simulink model "PlanerizerTest03"  (R2023a)
settings: Solver=FixedStepAuto  StartTime=0.0  StopTime=inf  FixedStep=0.005  RelTol=1e-3
libraries: speedgoatlib_IO691 x6, canmsglib x6, slrealtimeutilitieslib x2
settings Model: SimulationMode=external  NumberOfSteps=2  ExtModeEnableFloating=off  Creator=celwe  LastModifiedBy=johna
settings SolverCC: ConcurrentTasks=on  PositivePriorityOrder=on
settings OptimizationCC: BlockReduction=off  OptimizeBlockIOStorage=off
settings DebuggingCC: TasksWithSamePriorityMsg=none  UnconnectedInputMsg=warning  UnconnectedOutputMsg=warning  UnconnectedLineMsg=warning
settings HardwareCC: ProdBitPerLong=64  ProdLongLongMode=on  ProdHWDeviceType=Intel->x86-64 (Linux 64)
settings ModelReferenceCC: EnableRefExpFcnMdlSchedulingChecks=on
settings RTWCC: Description=Simulink Real-Time  SystemTargetFile=slrealtime.tlc  TemplateMakefile=slrealtime_default_tmf  Toolchain=Simulink Real-Time Toolchain  BuildConfiguration=Faster Runs  CodeExecutionProfiling=on  TargetLang=C++  DLArmComputeVersion=19.05

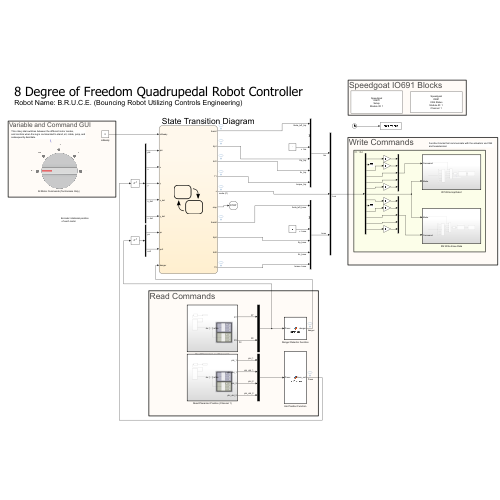
[thumbnail: Simulink's stored preview of the top-level diagram]
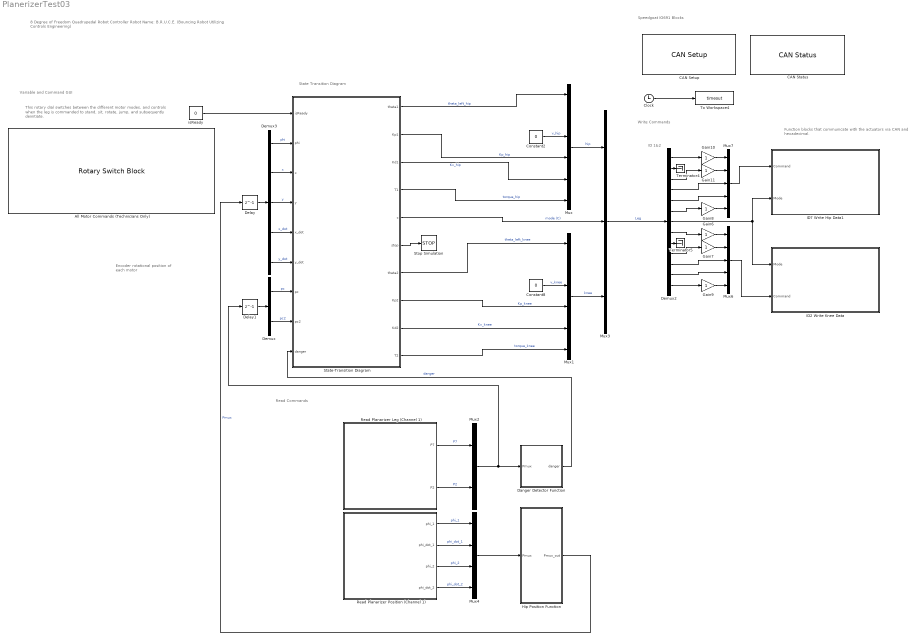
== system PlanerizerTest03 ==
  note: Variable and Command GUI
  note: 8 Degree of Freedom Quadrupedal Robot Controller
      | Robot Name: B.R.U.C.E. (Bouncing Robot Utilizing Controls Engineering)
  note: Encoder rotational position
      |  of each motor
  note: This rotary dial switches between the different motor modes,
      | and controls when the leg is commanded to stand, sit, rotate, jump, and
      | subsequently deinitiate.
  note: ID 1&2
  note: Function blocks that communicate with the actuators via CAN
      | and hexadecimal.
  note: Speedgoat IO691 Blocks
  note: Read Commands
  note: Write Commands
  note: State Transition Diagram
  "All Motor Commands (Technicians Only) " : RotarySwitchBlock
      settings: Values={{'Zeroing', 'Initiated', 'Stand', 'Sit', 'deinit'}, [0 1 2 3 4]}
  "CAN Setup " : speedgoatlib_IO691/Legacy/CAN Setup   moduletype=IO691  id=1  pciSlot=-1  chn1=CAN (HS)  chn2=CAN (HS)  chn3=Disabled  chn4=Disabled  initStruct=[]  termStruct=[]  ArbitrationbdrChn1=1.0 MBaud  ArbitrationManbdrChn1=[2,8,31,8]  FdbdrChn1=5.0 MBaud  FdManbdrChn1=[2,2,5,2]  ArbitrationbdrChn2=1.0 MBaud  ArbitrationManbdrChn2=[2,8,31,8]  FdbdrChn2=5.0 MBaud  FdManbdrChn2=[2,2,5,2]  ArbitrationbdrChn3=1.0 MBaud  ArbitrationManbdrChn3=[2,8,31,8]  FdbdrChn3=5.0 MBaud  FdManbdrChn3=[2,2,5,2]  ArbitrationbdrChn4=1.0 MBaud  ArbitrationManbdrChn4=[2,8,31,8]  FdbdrChn4=5.0 MBaud  FdManbdrChn4=[2,2,5,2]  moduleInitValues=[691 1 -1 -1]
      settings: SourceProductName=Simulink Real-Time: Speedgoat I/O Blockset
  CAN Status : speedgoatlib_IO691/Legacy/CAN Status  moduleId=1  sampleTime=-1  channel=1  busRecovery=Off  arrayOutput=off  controllerCpuLoad=off  controllerLiveCount=off  initModeAct=off  avgBusLoad=off  receiving=off  RxQueueEmpty=off  dataOverrunRcv=off  rxBufferLevel=off  txPending=off  dataOverrunTx=off  txBufferLevel=off  errWarnLimit=off  errPassLimit=off  errBusOff=off  busRecoveryCounter=off  busCouplingErr=off  transceiverErr=off  opMode=off  brp=off  timeSegment1=off  timeSegment2=off  synchronisationJumpWidth=off  dataTSEG1=off  dataTSEG2=off  dataSJW=off  moduleType=691  qtyStatBlk=1  ptIdx=0  isFDMod=0
      settings: SourceProductName=Simulink Real-Time: Speedgoat I/O Blockset
  Clock : Clock
  Constant2 : Constant  Value=0
  Constant8 : Constant  Value=0
  Danger Detector Function : MATLAB Function  TreatAsAtomicUnit=on
  Delay : Delay  DelayLength=1
  Delay1 : Delay  DelayLength=1
  Demux : Demux  Outputs=2
  Demux2 : Demux  Outputs=13
  Demux3 : Demux  Outputs=5
  Gain{6..11} (6 alike) : Gain
  Hip Position Function : MATLAB Function  TreatAsAtomicUnit=on
  ID2 Write Knee Data : Subsystem  TreatAsAtomicUnit=on
  ID7 Write Hip Data1 : Subsystem  TreatAsAtomicUnit=on
  Mux : Mux  Inputs=6
  Mux1 : Mux  Inputs=6
  Mux2 : Mux  Inputs=2
  Mux3 : Mux  Inputs=3
  Mux4 : Mux
  Mux6 : Mux  Inputs=5
  Mux7 : Mux  Inputs=5
  Read Planarizer Leg (Channel 1) : Subsystem  TreatAsAtomicUnit=on
  Read Planarizer Position (Channel 1) : Subsystem  TreatAsAtomicUnit=on
  State-Transition Diagram : Stateflow chart  TreatAsAtomicUnit=on
      settings: PortSchema="{\"entries\":[{\"content\":{\"sides\":[{\"content\":{\"connectorIds\":[\"In9\",\"In2\",\"In3\",\"In4\",\"In5\",\"In6\",\"In1\",\"In7\",\"In8\"]},\"type\":\"ConnectorPlacement.EquallySpacedRectSide\",\"uuid\":\"09499f21-f50c-4ce4-914e-8b9942bcc246\"},{\"content\":{\"connectorIds\":[\"Out2\",\"Out7\",\"Out9\",\"Out5\",\"Out4\",\"Out1\",\"Out3\",\"Out8\",\"Out10\",\"Out6\"],\"side\":\"RIGHT\"},\"type\":\"ConnectorPlacement.EquallySpacedRectSide\",\"uuid\":\"b935e908-ace3-4dfb-ad6d-08dfed6ffdb3\"},{\"content\":{\"side\":\"TOP\"},\"type\":\"ConnectorPlacement.EquallySpacedRectSide\",\"uuid\":\"4cd7c5d6-1f1f-4a1f-84b4-9b198395645e\"}]},\"type\":\"ConnectorPlacement.EquallySpacedConnector\",\"uuid\":\"2dc6a8af-05a8-4f21-87ab-6863f156f450\"}],\"packageUris\":[\"http://schema.mathworks.com/mf0/Connector/R2020b\"],\"version\":\"1.0\"}"
  Stop Simulation : Stop
  Terminator4 : Terminator
  Terminator5 : Terminator
  To Workspace4 : ToWorkspace  VariableName=timeout  SampleTime=-1
  isReady : Constant  Value=0
  wires:
  Mux/1 -> Mux3/1  "hip"
  State-Transition Diagram/7(Kp1) -> Mux/4  "Kp_hip"
  State-Transition Diagram/5(T1) -> Mux/6  "torque_hip"
  Constant8/1 -> Mux1/3  "v_knee"
  Mux1/1 -> Mux3/3  "knee"
  State-Transition Diagram/4(c) -> Mux3/2  "mode (C)"
  Mux2/1 -> Delay1/1, Danger Detector Function/1(Pmux)
  State-Transition Diagram/1(stop) -> Stop Simulation/1
  isReady/1 -> State-Transition Diagram/9(isReady)
  Clock/1 -> To Workspace4/1
  State-Transition Diagram/9(Kd1) -> Mux/5  "Kv_hip"
  Constant2/1 -> Mux/3  "v_hip"
  State-Transition Diagram/2(theta1) -> Mux/1  "theta_left_hip"
  Mux3/1 -> Demux2/1  "Leg"
  Mux7/1 -> ID7 Write Hip Data1/1(Command)
  Mux6/1 -> ID2 Write Knee Data/2(Command)
  Read Planarizer Leg (Channel 1)/2(P2) -> Mux2/2  "P2"
  Demux/2 -> State-Transition Diagram/7(pc2)  "pc2"
  Demux/1 -> State-Transition Diagram/1(pc)  "pc"
  Demux2/7 -> ID7 Write Hip Data1/2(Mode), ID2 Write Knee Data/1(Mode)
  Demux2/4 -> Mux7/3
  Demux2/10 -> Gain7/1
  Demux2/6 -> Gain8/1
  Demux2/5 -> Mux7/4
  Demux2/11 -> Mux6/3
  Demux2/3 -> Gain11/1
  Demux2/12 -> Mux6/4
  Gain11/1 -> Mux7/2
  Gain10/1 -> Mux7/1
  Gain7/1 -> Mux6/2
  Demux2/13 -> Gain9/1
  Gain9/1 -> Mux6/5
  Gain8/1 -> Mux7/5
  Gain6/1 -> Mux6/1
  State-Transition Diagram/3(theta2) -> Mux1/1  "theta_left_knee"
  State-Transition Diagram/10(Kd2) -> Mux1/5  "Kv_knee"
  State-Transition Diagram/6(T2) -> Mux1/6  "torque_knee"
  State-Transition Diagram/8(Kp2) -> Mux1/4  "Kp_knee"
  Read Planarizer Leg (Channel 1)/1(P7) -> Mux2/1  "P7"
  Danger Detector Function/1(danger) -> State-Transition Diagram/8(danger)  "danger"
  Demux2/2 -> Terminator4/1
  Demux2/1 -> Gain10/1
  Demux2/9 -> Terminator5/1
  Demux2/8 -> Gain6/1
  Read Planarizer Position (Channel 1)/1(phi_1) -> Mux4/1  "phi_1"
  Read Planarizer Position (Channel 1)/2(phi_dot_1) -> Mux4/2  "phi_dot_1"
  Read Planarizer Position (Channel 1)/3(phi_2) -> Mux4/3  "phi_2"
  Read Planarizer Position (Channel 1)/4(phi_dot_2) -> Mux4/4  "phi_dot_2"
  Mux4/1 -> Hip Position Function/1(Pmux)
  Hip Position Function/1(Pmux_out) -> Delay/1  "Pmux"
  Demux3/1 -> State-Transition Diagram/2(phi)  "phi"
  Demux3/2 -> State-Transition Diagram/3(x)  "x"
  Demux3/3 -> State-Transition Diagram/4(y)  "y"
  Demux3/4 -> State-Transition Diagram/5(x_dot)  "x_dot"
  Demux3/5 -> State-Transition Diagram/6(y_dot)  "y_dot"
  Delay/1 -> Demux3/1
  Delay1/1 -> Demux/1

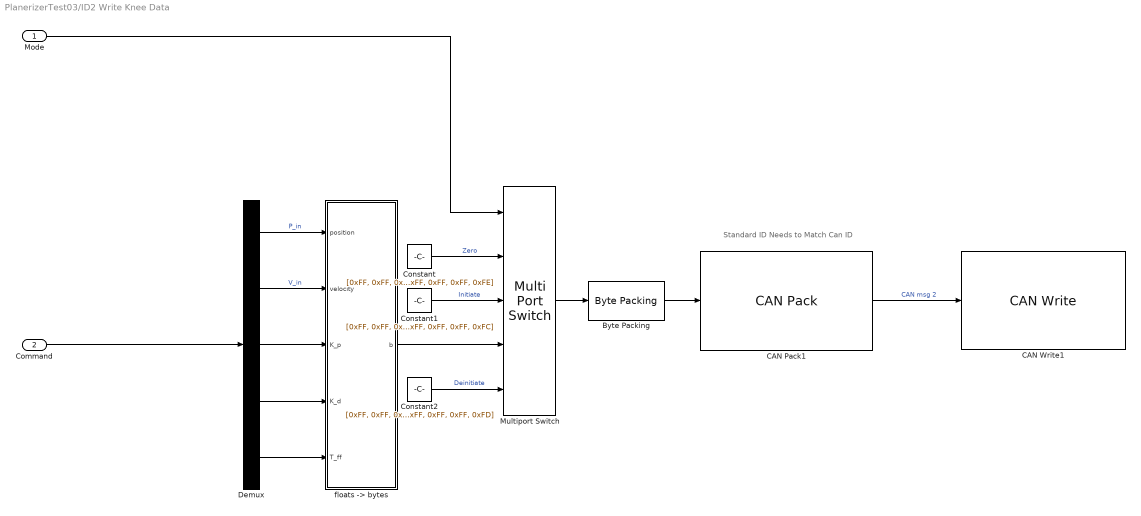
== system PlanerizerTest03/ID2 Write Knee Data ==
  note: Standard ID Needs to Match Can ID
  Mode : Inport
  Command : Inport  Port=2
  Byte Packing : slrealtimeutilitieslib/Byte Packing  MaskPackedDataType=uint8  MaskUnpackedDataTypes={['uint8']}  MaskAlignment=1
  CAN Pack1 : canmsglib/CAN Pack  MsgList=(none)  MsgName=CAN Msg  MsgIDType=Standard (11-bit identifier)  MsgIdentifier=2  MsgLength=8  Remote=off  ApplyMinMax=off  BusOutput=off  SignalInfo={ 'b1', '0', '8', 'LE', 'unsigned', 'Standard', '0', '1', '0', '-Inf', 'Inf'; 'b2', '8', '8', 'LE', 'unsigned', 'Standard', '0', '1', '0', '-Inf', 'Inf'; 'b3', '16', '8', 'LE', 'unsigned', 'Standard', '0', '1', '0', '-Inf', 'Inf'; 'b4', '24', '8', 'LE', 'unsigned', 'Standard', '0', '1', '0', '-Inf', 'Inf'; 'b5', '32', '8', 'LE', 'unsigned', 'Standard', '0', '1', '0', '-Inf', 'Inf'; 'b6', '40', '8', 'LE', 'unsigned', 'Standard', '0', '1', '0', '-Inf', 'Inf'; 'b7', '48', '8', 'LE', 'unsigned', 'Standard', '0', '1', '0', '-Inf', 'Inf'; 'b8', '56', '8', 'LE', 'unsigned', 'Standard', '0', '1', '0', '-Inf', 'Inf' }
      settings: DataFormat=raw data
  CAN Write1 : speedgoatlib_IO691/Legacy/CAN Write  id=1  ts=-1  channel=1  messageType=CAN  BusInput=off  enableStatusPort=off  canType=CAN (HS)  initValues=[691 1 -1 0 1 1 0 0]
      settings: SourceProductName=Simulink Real-Time: Speedgoat I/O Blockset
  Constant : Constant  Value=[0xFF, 0xFF, 0xFF, 0xFF, 0xFF, 0xFF, 0xFF, 0xFE]
  Constant1 : Constant  Value=[0xFF, 0xFF, 0xFF, 0xFF, 0xFF, 0xFF, 0xFF, 0xFC]
  Constant2 : Constant  Value=[0xFF, 0xFF, 0xFF, 0xFF, 0xFF, 0xFF, 0xFF, 0xFD]
  Demux : Demux  Outputs=5
  Multiport Switch : MultiPortSwitch  Inputs=4  DiagnosticForDefault=None  SaturateOnIntegerOverflow=off  InputSameDT=off
  "floats -> bytes" : MATLAB Function  TreatAsAtomicUnit=on
  wires:
  Demux/5 -> "floats -> bytes"/5(T_ff)
  Multiport Switch/1 -> Byte Packing/1
  Demux/4 -> "floats -> bytes"/4(K_d)
  Demux/1 -> "floats -> bytes"/1(position)  "P_in"
  Constant/1 -> Multiport Switch/2  "Zero"
  Demux/2 -> "floats -> bytes"/2(velocity)  "V_in"
  Constant2/1 -> Multiport Switch/5  "Deinitiate"
  CAN Pack1/1 -> CAN Write1/1  "CAN msg 2"
  Byte Packing/1 -> CAN Pack1/1
  Constant1/1 -> Multiport Switch/3  "Initiate"
  "floats -> bytes"/1(b) -> Multiport Switch/4
  Demux/3 -> "floats -> bytes"/3(K_p)
  Mode/1 -> Multiport Switch/1
  Command/1 -> Demux/1

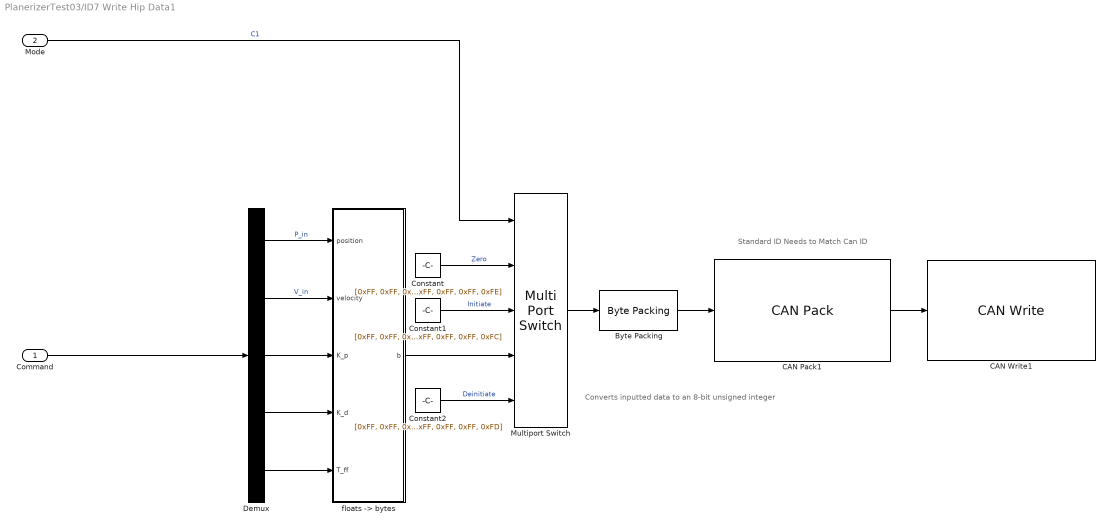
== system PlanerizerTest03/ID7 Write Hip Data1 ==
  note: Standard ID Needs to Match Can ID
  note: Converts inputted data to an 8-bit unsigned integer
  Command : Inport
  Mode : Inport  Port=2
  Byte Packing : slrealtimeutilitieslib/Byte Packing  MaskPackedDataType=uint8  MaskUnpackedDataTypes={['uint8']}  MaskAlignment=1
  CAN Pack1 : canmsglib/CAN Pack  MsgList=(none)  MsgName=CAN Msg  MsgIDType=Standard (11-bit identifier)  MsgIdentifier=7  MsgLength=8  Remote=off  ApplyMinMax=off  BusOutput=off  SignalInfo={ 'b1', '0', '8', 'LE', 'unsigned', 'Standard', '0', '1', '0', '-Inf', 'Inf'; 'b2', '8', '8', 'LE', 'unsigned', 'Standard', '0', '1', '0', '-Inf', 'Inf'; 'b3', '16', '8', 'LE', 'unsigned', 'Standard', '0', '1', '0', '-Inf', 'Inf'; 'b4', '24', '8', 'LE', 'unsigned', 'Standard', '0', '1', '0', '-Inf', 'Inf'; 'b5', '32', '8', 'LE', 'unsigned', 'Standard', '0', '1', '0', '-Inf', 'Inf'; 'b6', '40', '8', 'LE', 'unsigned', 'Standard', '0', '1', '0', '-Inf', 'Inf'; 'b7', '48', '8', 'LE', 'unsigned', 'Standard', '0', '1', '0', '-Inf', 'Inf'; 'b8', '56', '8', 'LE', 'unsigned', 'Standard', '0', '1', '0', '-Inf', 'Inf' }
      settings: DataFormat=raw data
  CAN Write1 : speedgoatlib_IO691/Legacy/CAN Write  id=1  ts=-1  channel=1  messageType=CAN  BusInput=off  enableStatusPort=off  canType=CAN (HS)  initValues=[691 1 -1 0 1 1 0 0]
      settings: SourceProductName=Simulink Real-Time: Speedgoat I/O Blockset
  Constant : Constant  Value=[0xFF, 0xFF, 0xFF, 0xFF, 0xFF, 0xFF, 0xFF, 0xFE]
  Constant1 : Constant  Value=[0xFF, 0xFF, 0xFF, 0xFF, 0xFF, 0xFF, 0xFF, 0xFC]
  Constant2 : Constant  Value=[0xFF, 0xFF, 0xFF, 0xFF, 0xFF, 0xFF, 0xFF, 0xFD]
  Demux : Demux  Outputs=5
  Multiport Switch : MultiPortSwitch  Inputs=4  DiagnosticForDefault=None  SaturateOnIntegerOverflow=off  InputSameDT=off
  "floats -> bytes" : MATLAB Function  TreatAsAtomicUnit=on
  wires:
  Demux/5 -> "floats -> bytes"/5(T_ff)
  Multiport Switch/1 -> Byte Packing/1
  Demux/4 -> "floats -> bytes"/4(K_d)
  Demux/1 -> "floats -> bytes"/1(position)  "P_in"
  Constant/1 -> Multiport Switch/2  "Zero"
  Demux/2 -> "floats -> bytes"/2(velocity)  "V_in"
  Constant2/1 -> Multiport Switch/5  "Deinitiate"
  CAN Pack1/1 -> CAN Write1/1
  Byte Packing/1 -> CAN Pack1/1
  Constant1/1 -> Multiport Switch/3  "Initiate"
  "floats -> bytes"/1(b) -> Multiport Switch/4
  Demux/3 -> "floats -> bytes"/3(K_p)
  Mode/1 -> Multiport Switch/1  "C1"
  Command/1 -> Demux/1

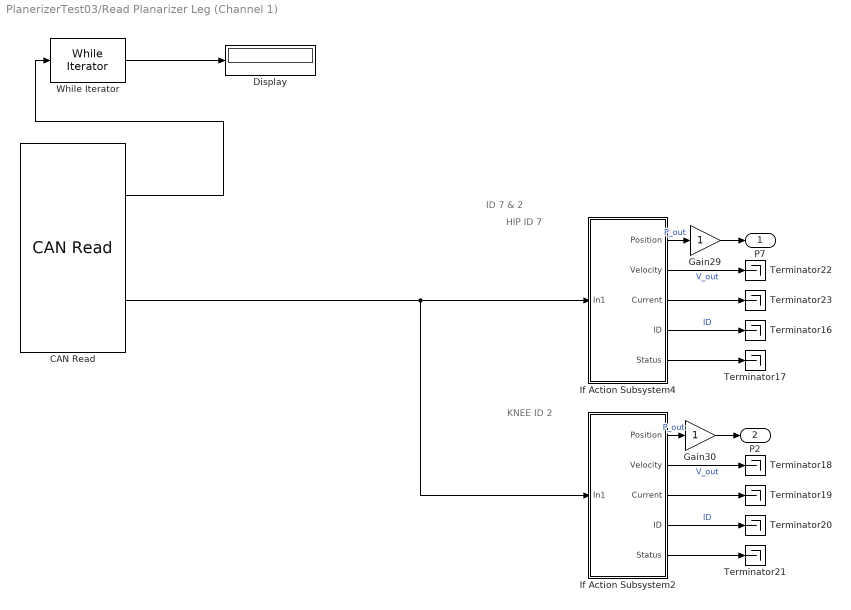
== system PlanerizerTest03/Read Planarizer Leg (Channel 1) ==
  note: KNEE ID 2
  note: HIP ID 7
  note: ID 7 & 2
  CAN Read : speedgoatlib_IO691/Legacy/CAN Read  id=1  ts=-1  channel=1  messageType=CAN  canType=CAN (HS)  BusOutput=off  initValues=[691 1 -1 0 1 1 0]
      settings: SourceProductName=Simulink Real-Time: Speedgoat I/O Blockset
  Display : Display
  Gain29 : Gain
  Gain30 : Gain
  If Action Subsystem2 : Subsystem  TreatAsAtomicUnit=on
  If Action Subsystem4 : Subsystem  TreatAsAtomicUnit=on
  Terminator{16..23} (8 alike) : Terminator
  While Iterator : WhileIterator  MaxIters=-1  WhileBlockType=do-while  ResetStates=reset  ShowIterationPort=on
  P7 : Outport
  P2 : Outport  Port=2
  wires:
  CAN Read/1 -> While Iterator/1
  While Iterator/1 -> Display/1
  CAN Read/2 -> If Action Subsystem2/1(In1), If Action Subsystem4/1(In1)
  Gain30/1 -> P2/1
  If Action Subsystem2/1(Position) -> Gain30/1  "P_out"
  If Action Subsystem2/4(ID) -> Terminator20/1  "ID"
  If Action Subsystem4/4(ID) -> Terminator16/1  "ID"
  Gain29/1 -> P7/1
  If Action Subsystem4/1(Position) -> Gain29/1  "P_out"
  If Action Subsystem2/2(Velocity) -> Terminator18/1  "V_out"
  If Action Subsystem4/3(Current) -> Terminator23/1
  If Action Subsystem4/5(Status) -> Terminator17/1
  If Action Subsystem2/3(Current) -> Terminator19/1
  If Action Subsystem2/5(Status) -> Terminator21/1
  If Action Subsystem4/2(Velocity) -> Terminator22/1  "V_out"

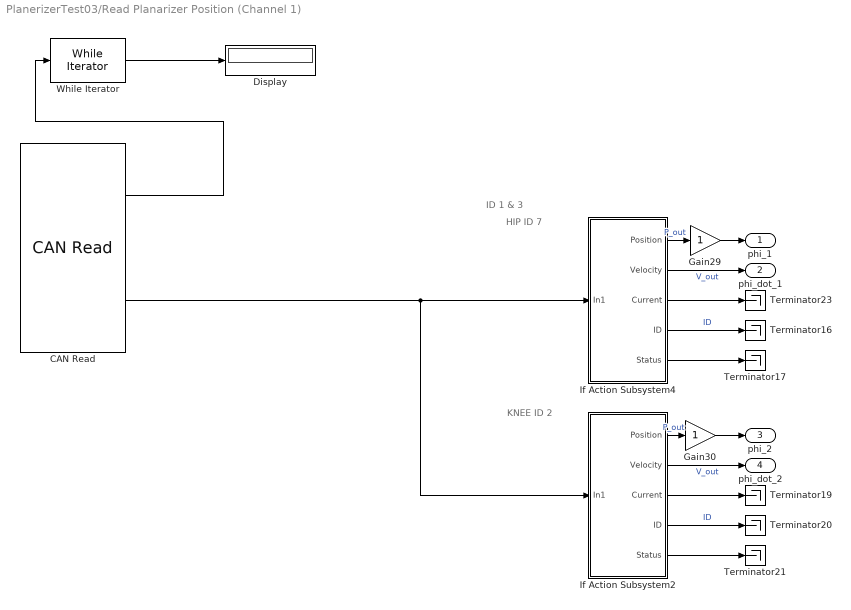
== system PlanerizerTest03/Read Planarizer Position (Channel 1) ==
  note: KNEE ID 2
  note: HIP ID 7
  note: ID 1 & 3
  CAN Read : speedgoatlib_IO691/Legacy/CAN Read  id=1  ts=-1  channel=1  messageType=CAN  canType=CAN (HS)  BusOutput=off  initValues=[691 1 -1 0 1 1 0]
      settings: SourceProductName=Simulink Real-Time: Speedgoat I/O Blockset
  Display : Display
  Gain29 : Gain
  Gain30 : Gain
  If Action Subsystem2 : Subsystem  TreatAsAtomicUnit=on
  If Action Subsystem4 : Subsystem  TreatAsAtomicUnit=on
  Terminator{16..17,19..21,23} (6 alike) : Terminator
  While Iterator : WhileIterator  MaxIters=-1  WhileBlockType=do-while  ResetStates=reset  ShowIterationPort=on
  phi_1 : Outport
  phi_dot_1 : Outport  Port=2
  phi_2 : Outport  Port=3
  phi_dot_2 : Outport  Port=4
  wires:
  CAN Read/1 -> While Iterator/1
  While Iterator/1 -> Display/1
  CAN Read/2 -> If Action Subsystem2/1(In1), If Action Subsystem4/1(In1)
  If Action Subsystem2/1(Position) -> Gain30/1  "P_out"
  If Action Subsystem2/4(ID) -> Terminator20/1  "ID"
  If Action Subsystem4/4(ID) -> Terminator16/1  "ID"
  Gain29/1 -> phi_1/1
  If Action Subsystem4/1(Position) -> Gain29/1  "P_out"
  If Action Subsystem2/2(Velocity) -> phi_dot_2/1  "V_out"
  If Action Subsystem4/3(Current) -> Terminator23/1
  If Action Subsystem4/5(Status) -> Terminator17/1
  If Action Subsystem2/3(Current) -> Terminator19/1
  If Action Subsystem2/5(Status) -> Terminator21/1
  If Action Subsystem4/2(Velocity) -> phi_dot_1/1  "V_out"
  Gain30/1 -> phi_2/1

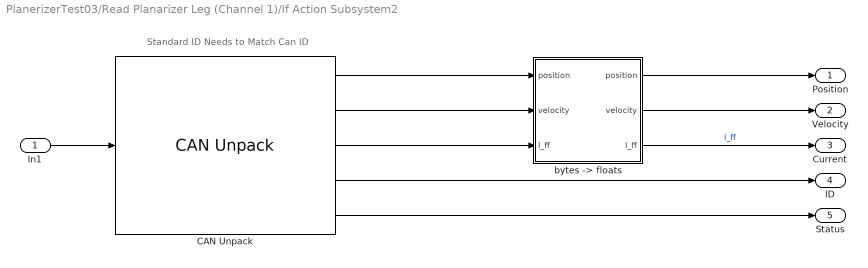
== system PlanerizerTest03/Read Planarizer Leg (Channel 1)/If Action Subsystem2 ==
  note: Standard ID Needs to Match Can ID
  In1 : Inport
  CAN Unpack : canmsglib/CAN Unpack  MsgList=(none)  MsgName=CAN Msg  MsgIDType=Standard (11-bit identifier)  MsgIdentifier=2  MsgLength=6  SignalInfo={ 'position', '16', '16', 'BE', 'unsigned', 'Standard', '0', '1', '0', '0', '65535'; 'velocity', '36', '12', 'BE', 'unsigned', 'Standard', '0', '1', '0', '0', '4095'; 'current', '40', '12', 'BE', 'unsigned', 'Standard', '0', '1', '0', '0', '4095'; 'id', '0', '8', 'BE', 'unsigned', 'Standard', '0', '1', '0', '0', '255' }  IDPort=off  TimestampPort=off  ErrorPort=off  RemotePort=off  LengthPort=off  StatusPort=on  ApplyMinMax=off
  "bytes -> floats" : MATLAB Function  TreatAsAtomicUnit=on
  Position : Outport
  Velocity : Outport  Port=2
  Current : Outport  Port=3
  ID : Outport  Port=4
  Status : Outport  Port=5
  wires:
  CAN Unpack/5 -> Status/1
  CAN Unpack/1 -> "bytes -> floats"/1("position ")
  CAN Unpack/3 -> "bytes -> floats"/3("I_ff ")
  "bytes -> floats"/1(position) -> Position/1
  CAN Unpack/4 -> ID/1
  "bytes -> floats"/2(velocity) -> Velocity/1
  "bytes -> floats"/3(I_ff) -> Current/1  "I_ff"
  CAN Unpack/2 -> "bytes -> floats"/2("velocity ")
  In1/1 -> CAN Unpack/1

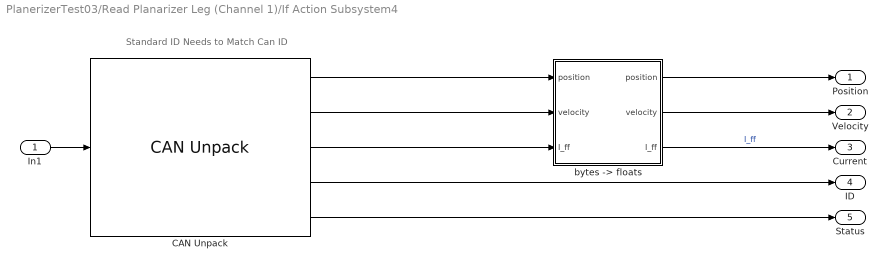
== system PlanerizerTest03/Read Planarizer Leg (Channel 1)/If Action Subsystem4 ==
  note: Standard ID Needs to Match Can ID
  In1 : Inport
  CAN Unpack : canmsglib/CAN Unpack  MsgList=(none)  MsgName=CAN Msg  MsgIDType=Standard (11-bit identifier)  MsgIdentifier=7  MsgLength=6  SignalInfo={ 'position', '16', '16', 'BE', 'unsigned', 'Standard', '0', '1', '0', '0', '65535'; 'velocity', '36', '12', 'BE', 'unsigned', 'Standard', '0', '1', '0', '0', '4095'; 'current', '40', '12', 'BE', 'unsigned', 'Standard', '0', '1', '0', '0', '4095'; 'id', '0', '8', 'BE', 'unsigned', 'Standard', '0', '1', '0', '0', '255' }  IDPort=off  TimestampPort=off  ErrorPort=off  RemotePort=off  LengthPort=off  StatusPort=on  ApplyMinMax=off
  "bytes -> floats" : MATLAB Function  TreatAsAtomicUnit=on
  Position : Outport
  Velocity : Outport  Port=2
  Current : Outport  Port=3
  ID : Outport  Port=4
  Status : Outport  Port=5
  wires:
  CAN Unpack/5 -> Status/1
  CAN Unpack/3 -> "bytes -> floats"/3("I_ff ")
  CAN Unpack/4 -> ID/1
  "bytes -> floats"/2(velocity) -> Velocity/1
  "bytes -> floats"/3(I_ff) -> Current/1  "I_ff"
  CAN Unpack/2 -> "bytes -> floats"/2("velocity ")
  In1/1 -> CAN Unpack/1
  CAN Unpack/1 -> "bytes -> floats"/1("position ")
  "bytes -> floats"/1(position) -> Position/1

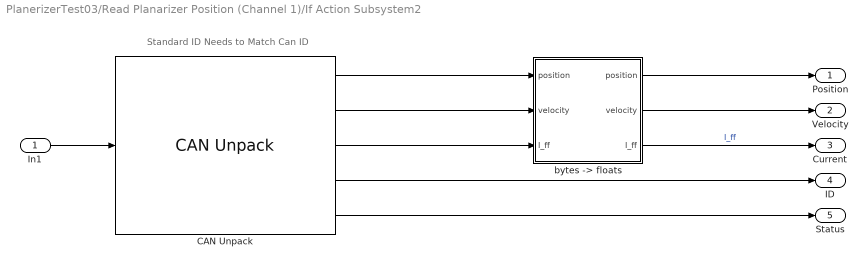
== system PlanerizerTest03/Read Planarizer Position (Channel 1)/If Action Subsystem2 ==
  note: Standard ID Needs to Match Can ID
  In1 : Inport
  CAN Unpack : canmsglib/CAN Unpack  MsgList=(none)  MsgName=CAN Msg  MsgIDType=Standard (11-bit identifier)  MsgIdentifier=2  MsgLength=6  SignalInfo={ 'position', '16', '16', 'BE', 'unsigned', 'Standard', '0', '1', '0', '0', '65535'; 'velocity', '36', '12', 'BE', 'unsigned', 'Standard', '0', '1', '0', '0', '4095'; 'current', '40', '12', 'BE', 'unsigned', 'Standard', '0', '1', '0', '0', '4095'; 'id', '0', '8', 'BE', 'unsigned', 'Standard', '0', '1', '0', '0', '255' }  IDPort=off  TimestampPort=off  ErrorPort=off  RemotePort=off  LengthPort=off  StatusPort=on  ApplyMinMax=off
  "bytes -> floats" : MATLAB Function  TreatAsAtomicUnit=on
  Position : Outport
  Velocity : Outport  Port=2
  Current : Outport  Port=3
  ID : Outport  Port=4
  Status : Outport  Port=5
  wires:
  CAN Unpack/5 -> Status/1
  CAN Unpack/1 -> "bytes -> floats"/1("position ")
  CAN Unpack/3 -> "bytes -> floats"/3("I_ff ")
  "bytes -> floats"/1(position) -> Position/1
  CAN Unpack/4 -> ID/1
  "bytes -> floats"/2(velocity) -> Velocity/1
  "bytes -> floats"/3(I_ff) -> Current/1  "I_ff"
  CAN Unpack/2 -> "bytes -> floats"/2("velocity ")
  In1/1 -> CAN Unpack/1

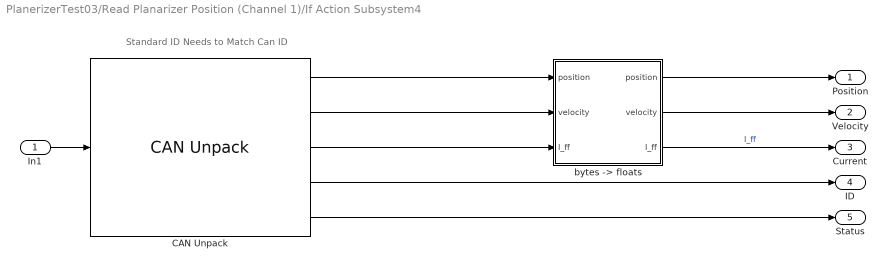
== system PlanerizerTest03/Read Planarizer Position (Channel 1)/If Action Subsystem4 ==
  note: Standard ID Needs to Match Can ID
  In1 : Inport
  CAN Unpack : canmsglib/CAN Unpack  MsgList=(none)  MsgName=CAN Msg  MsgIDType=Standard (11-bit identifier)  MsgIdentifier=7  MsgLength=6  SignalInfo={ 'position', '16', '16', 'BE', 'unsigned', 'Standard', '0', '1', '0', '0', '65535'; 'velocity', '36', '12', 'BE', 'unsigned', 'Standard', '0', '1', '0', '0', '4095'; 'current', '40', '12', 'BE', 'unsigned', 'Standard', '0', '1', '0', '0', '4095'; 'id', '0', '8', 'BE', 'unsigned', 'Standard', '0', '1', '0', '0', '255' }  IDPort=off  TimestampPort=off  ErrorPort=off  RemotePort=off  LengthPort=off  StatusPort=on  ApplyMinMax=off
  "bytes -> floats" : MATLAB Function  TreatAsAtomicUnit=on
  Position : Outport
  Velocity : Outport  Port=2
  Current : Outport  Port=3
  ID : Outport  Port=4
  Status : Outport  Port=5
  wires:
  CAN Unpack/5 -> Status/1
  CAN Unpack/3 -> "bytes -> floats"/3("I_ff ")
  CAN Unpack/4 -> ID/1
  "bytes -> floats"/2(velocity) -> Velocity/1
  "bytes -> floats"/3(I_ff) -> Current/1  "I_ff"
  CAN Unpack/2 -> "bytes -> floats"/2("velocity ")
  In1/1 -> CAN Unpack/1
  CAN Unpack/1 -> "bytes -> floats"/1("position ")
  "bytes -> floats"/1(position) -> Position/1

== matlab function PlanerizerTest03/Read Planarizer Leg (Channel 1)/If Action Subsystem4/bytes -> floats ==
  data: position input; position output; velocity output; I_ff output; velocity input; I_ff input
function [position, velocity, I_ff] = fcn(position, velocity, I_ff)

P_MIN  =-95.5;  % [rad]
P_MAX  = 95.5;  % [rad]
V_MIN  =-45;    % [rad/s]
V_MAX  = 45;    % [rad/s]
I_MIN  =-40;    % []
I_MAX  = 40;    % []

position = position*(P_MAX  - P_MIN)/65535+ P_MIN;
velocity = velocity*(V_MAX  - V_MIN)/4095 + V_MIN;
I_ff     = I_ff*(I_MAX  - I_MIN)/4095 + I_MIN;

== matlab function PlanerizerTest03/Read Planarizer Leg (Channel 1)/If Action Subsystem2/bytes -> floats ==
  data: position input; position output; velocity output; I_ff output; velocity input; I_ff input
function [position, velocity, I_ff] = fcn(position, velocity, I_ff)

P_MIN  =-95.5;  % [rad]
P_MAX  = 95.5;  % [rad]
V_MIN  =-45;    % [rad/s]
V_MAX  = 45;    % [rad/s]
I_MIN  =-40;    % []
I_MAX  = 40;    % []

position = position*(P_MAX  - P_MIN)/65535+ P_MIN;
velocity = velocity*(V_MAX  - V_MIN)/4095 + V_MIN;
I_ff     = I_ff*(I_MAX  - I_MIN)/4095 + I_MIN;

== matlab function PlanerizerTest03/Read Planarizer Position (Channel 1)/If Action Subsystem2/bytes -> floats ==
  data: position input; position output; velocity output; I_ff output; velocity input; I_ff input
function [position, velocity, I_ff] = fcn(position, velocity, I_ff)

P_MIN  =-95.5;  % [rad]
P_MAX  = 95.5;  % [rad]
V_MIN  =-45;    % [rad/s]
V_MAX  = 45;    % [rad/s]
I_MIN  =-40;    % []
I_MAX  = 40;    % []

position = position*(P_MAX  - P_MIN)/65535+ P_MIN;
velocity = velocity*(V_MAX  - V_MIN)/4095 + V_MIN;
I_ff     = I_ff*(I_MAX  - I_MIN)/4095 + I_MIN;

== matlab function PlanerizerTest03/ID7 Write Hip Data1/floats -> bytes ==
  data: position input; b output uint8 size=8; velocity input; K_p input; K_d input; T_ff input
function b = fcn(position, velocity, K_p, K_d, T_ff)

P_MIN  =-95.5;  % [rad]
P_MAX  = 95.5;  % [rad]
V_MIN  =-45;    % [rad/s] 30 to 45
V_MAX  = 45;    % [rad/s]
KP_MIN = 0;     % [Nm/rad]
KP_MAX = 500;   % [Nm/rad]
KD_MIN = 0;     % [Nm*s/rad
KD_MAX = 5;     % [Nm*s/rad
T_MIN  =-18;    % [Nm]
T_MAX  = 18;    % [Nm]

position = floor((max(min(position,P_MAX) ,P_MIN)  - P_MIN )*65535/(P_MAX  - P_MIN));
velocity = floor((max(min(velocity,V_MAX) ,V_MIN)  - V_MIN )*4095 /(V_MAX  - V_MIN));
K_p      = floor((max(min(K_p     ,KP_MAX),KP_MIN) - KP_MIN)*4095 /(KP_MAX - KP_MIN));
K_d      = floor((max(min(K_d     ,V_MAX) ,V_MIN)  - KD_MIN)*4095 /(KD_MAX - KD_MIN));
T_ff     = floor((max(min(T_ff    ,V_MAX) ,V_MIN)  - T_MIN )*4095 /(T_MAX  - T_MIN));

p  = dec2bin(position);
p  = [repmat('0', 1, 16-length(p)),p];
v  = dec2bin(velocity);
v  = [repmat('0', 1, 12-length(v)),v];
kp = dec2bin(K_p);
kp  = [repmat('0', 1, 12-length(kp)),kp];
kd = dec2bin(K_d);
kd  = [repmat('0', 1, 12-length(kd)),kd];
t  = dec2bin(T_ff);
t  = [repmat('0', 1, 12-length(t)),t];

B = repmat('0', 8, 8);

B(1,:) = p(1:8);
B(2,:) = p(9:16);
B(3,:) = v(1:8);
B(4,:) = [v(9:12),kp(1:4)];
B(5,:) = kp(5:12);
B(6,:) = kd(1:8);
B(7,:) = [kd(9:12),t(1:4)];
B(8,:) = t(5:12);

B  = bin2dec(B);

b = uint8(B);

== matlab function PlanerizerTest03/Read Planarizer Position (Channel 1)/If Action Subsystem4/bytes -> floats ==
  data: position input; position output; velocity output; I_ff output; velocity input; I_ff input
function [position, velocity, I_ff] = fcn(position, velocity, I_ff)

P_MIN  =-95.5;  % [rad]
P_MAX  = 95.5;  % [rad]
V_MIN  =-45;    % [rad/s]
V_MAX  = 45;    % [rad/s]
I_MIN  =-40;    % []
I_MAX  = 40;    % []

position = position*(P_MAX  - P_MIN)/65535+ P_MIN;
velocity = velocity*(V_MAX  - V_MIN)/4095 + V_MIN;
I_ff     = I_ff*(I_MAX  - I_MIN)/4095 + I_MIN;

== matlab function PlanerizerTest03/Danger Detector Function ==
  data: Pmux input; danger output
function danger = isDanger(Pmux)
    % Pmux position matrix radians
    %       [p(ID1),p(ID2),p(ID3),p(IDN)]

    
    p1Max = 2; 
    p1Min = -2;
    p2Max = 2;
    p2Min = -2;
    
    P1 = Pmux(1:2:end);
    P2 = Pmux(2:2:end);
       
    danger = 0;
    if((0<sum([P1>p1Max] + [P1<p1Min] - [P1<=-95.5])) || (0<sum([P2>p2Max] + [P2<p2Min] - [P2<=-95.5])))
    
%     if((0<sum([P1>p1Max] + [P1<p1Min])) || (0<sum([P2>p2Max] + [P2<p2Min])))
        danger = 1;
    end

== stateflow chart PlanerizerTest03/State-Transition Diagram ==
  state Start
  note: Simulink State Transition Diagram
      | "IsReady" is a user defined varable that controls the flow through the Finite State Mechine
      | Commands: 0. Zero
      | 1. Init
      | 2. Command
      | 4. Deinit
  state Zero
    entry:
    c = 1;
  state Init
    entry:
    c = 2;
  state SlowDown
    entry:
    %deinitiate mode
    c = 4
  state Command
    entry:
    c = 3;
    state Ideal
    state Stand
      entry:
      to = t;
      theta1 = pc;
      po1 = theta1;
      slope1 = (sp(1,1) - po1)/5;
      theta2 = pc2;
      po2 = theta2;
      slope2 = (sp(1,1) - po2)/5;
      during:
      theta1  = po1  + slope1*(t-to);
      theta2  = po2  + slope2*(t-to);
    state Stance
      entry:
      to = t;
      during:
      P = Phip(p,q);
      V = Vhip(p,q);
      tau_ff = FeedForwardTorque(p,u,Fd)
      % Hip y Position
      yd = p.yhipd
      ya = P(2)
      e_y = yd - ya
      % Hip x Velecity
      Vxd = p.Vxhipd
      Vxa = V(1)
      e_Vx = Vxd - Vxa
      % Hip y Velecity
      Vyd = p.Vyhipd
      Vya = V(2)
      e_Vy = Vyd - Vya
      % Compute error Matricies
      e = e_y
      ed = [e_Vx; e_Vy]
      tau = tau_ff + Kp_s*e + Kd_s*ed
    state Flight
      entry:
      to = t;
      during:
      thd = Traj(t,tf,C);
      % Position θ₁
      th1d = thd(1,1);
      th1a = q(1);
      e_th1 = th1d - th1a;
      % Position θ₃
      th3d = thd(1,2);
      th3a = q(2);
      e_th3 = th3d - th3a;
      e = [e_th1;e_th3];
      % Position Derivative, θ̇₁
      thd1d = thd(2,1);
      thd1a = q(5);
      ed_th1 = thd1d - thd1a;
      %  Position Derivative, θ̇₃
      thd3d = thd(2,2);
      thd3a = q(6);
      ed_th3 = thd3d - thd3a
      ed = [ed_th1;ed_th3]
      Tau = Kp_f*e + Kd_f*ed
    Ideal -> Stand
    (default) -> Ideal
    Stand -> (junction 297)
    Flight -> (junction 297)
    (junction 297) -> Stance
    Stance -> Flight
  state FinalShutdown
    entry:
    Kp1 = 0;
    Kp2 = 0;
    theta1 = 0;
    theta2 = 0;
    T1 = 0;
    T2 = 0;
    Kd1 = .1;
    Kd2 = .1;
  state Deinitiate
    entry:
    c = 4;
  (default) -> Start
  Start -> Init [order 2] : [isReady == 1]
  Start -> Zero [order 1] : [isReady == 0]
  SlowDown -> Zero [order 2] : [after(1,sec) & ~(pc == pc2) ]
  SlowDown -> Init [order 1] : [isReady == 1]
  Init -> FinalShutdown [order 2] : [isReady == 4 | danger == 1]
  Zero -> SlowDown
  Init -> Command [order 1] : [isReady == 2]
  Command -> FinalShutdown : [isReady == 4 | danger == 1]
  FinalShutdown -> Deinitiate
  Deinitiate -> (junction 36) : after(3,sec)
  (junction 36) -> Deinitiate : {stop = 1;}
  data: q function_input; Fxd function_input; tau_ff function_output; A function_input; w function_input; phi function_input; xo function_input; p function_input; A function_output; phi function_output; sp function_input; y_hop function_input; Vxhipd function_output; yhipd function_input; Vyhipd function_output; t function_input; tf function_input; C function_input; thd function_output; q function_input; tf function_input; sp function_input; C function_output; q function_input; sp function_input; t function_output; q function_input; sp function_input; t function_output; stop output =0; theta1 output; theta2 output; c output; pc input; phi input; x input; y input; x_dot input; y_dot input; pc2 input; T1 output =0; T2 output =0; Kp1 output =30; Kp2 output =30; Kd1 output =.2; Kd2 output =.2; danger input; isReady input
  function tau_ff = FeedForwardTorque(q,Fxd,A,w,phi):
    | function tau_ff = FeedForwardTorque(q,Fxd,A,w,phi)
    |     % Mass Constants
    |     m1 = 1;
    |     m2 = 1;
    |     % Length Constants
    |     LA = 1;
    |     LB = 1;
    |     L1 = LA/2;
    |     L2 = LB/2;
    |     % Damping Coefficents
    |     c1 = 2;
    |     c2 = 2;
    |     % Bar Mass Inertias
    |     I1 = 0.4167;
    |     I2 = 0.4167;
    |     % Gravity
    |     g = 10;
    | 
    |     F = [Fxd; A*sin(w*t + phi)];
    |     J = [LB*cos(q(1)+q(2)) + LA*cos(q(1))  LB*cos(q(1)+q(2));
    |         LB*sin(q(1)+q(2)) + LA*sin(q(1)  LB*sin(q(1)+q(2))];
    | 
    |    tau_mass = [m1*g*L1*sin(q(1)) + m2*g*(L2*sin(q(1)+q(2)) + LA*sin(q(1)));
    |              m2*g*L2*sin(q(1)+q(2))];
    | 
    |    tau_ff = -J'*F - tau_mass;
    | end
  function [A, phi] = APhiGRFCalc(xo,p):
    | function [A, phi] = APhiGRFCalc(xo,p)
    |     % Mass Constants
    |     m1 = 1;
    |     m2 = 1;
    |     % Length Constants
    |     LA = 1;
    |     LB = 1;
    |     L1 = LA/2;
    |     L2 = LB/2;
    |     % Damping Coefficents
    |     c1 = 2;
    |     c2 = 2;
    |     % Spring Parameter
    |     ks = 1001
    |     cs = 550
    |     % Gravity
    |     g = 10;
    | 
    |    u = Aug(p,x0,0)
    | 
    |    A = (((m1+m2)*w*(Vyhipd - u(8))^2 + (cs*u(10))^2)/((m1+m2)*w*(Vyhipd - u(8)));
    |    phi = asin(-cs*u(10)/A);
    | 
    | end
  function [Vxhipd,Vyhipd] = VhipCalc(sp,y_hop,yhipd):
    | function [Vxhipd,Vyhipd] = VhipCalc(sp,y_hop,yhipd)
    |     % Mass Constants
    |     m1 = 1;
    |     m2 = 1;
    |     % Length Constants
    |     LA = 1;
    |     LB = 1;
    |     L1 = LA/2;
    |     L2 = LB/2;
    |     % Damping Coefficents
    |     c1 = 2;
    |     c2 = 2;
    |     % Spring Parameter
    |     ks = 1001
    |     cs = 550
    |     % Gravity
    |     g = 10;
    | 
    |     yf = LA*cos(sp(1,1)) + LB*cos(sp(1,1)+sp(1,2))
    |     Vyhipd = sqrt(2*g*(y_hop-yhipd))
    |     Vxhipd = dx_hop*g/(Vyhipd + sqrt(Vyhipd^2 + 2*g*(yhipd - yf)))
    | end
  function thd = Traj(t,tf,C):
    | function thd = Traj(t,tf,C)
    | 
    |     if p.tf < t
    |         t = p.tf
    |     end
    |     
    |     thd = [1 t   t^2 t^3;
    |            0 1 2*t 3*t^2]*C
    | end
  function C = TrajPlan(q,tf,sp):
    | function C = TrajPlan(q,tf,sp)
    |     M_t =[1   0    0    0;
    |           0   1    0    0;
    |           1   tf   tf^2 tf^3;
    |           0   1    2*tf 3*tf^2];
    |     M_IC = [q(1:2)'; q(5:6)'; sp];
    |     C = (M_t^-1)*M_IC;
    | end
  function t = FlightTimeApprox(q,sp):
    | function t = FlightTimeApprox(q,sp)
    | 
    |     % Mass Constants
    |     m1 = 1;
    |     m2 = 1;
    |     % Length Constants
    |     LA = 1;
    |     LB = 1;
    |     L1 = LA/2;
    |     L2 = LB/2;
    |     % Damping Coefficents
    |     c1 = 2;
    |     c2 = 2;
    |     % Bar Mass Inertias
    |     I1 = 0.4167;
    |     I2 = 0.4167;
    |     % Gravity
    |     g = 10;
    | 
    |     yf = LA*cos(sp(1,1)) + LB*cos(sp(1,1)+sp(1,2));
    |     if((q(8)^2-2*g*(yf-q(4)))>=0)
    |         t = (q(8) + sqrt(q(8)^2-2*get*(yf-q(4))))/g;
    |     else
    |         t = 0.005;
    |     end
    | end
  function t = FlightTimeApprox1(q,sp):
    | function t = FlightTimeApprox1(q,sp)
    | 
    |     % Mass Constants
    |     m1 = 1;
    |     m2 = 1;
    |     % Length Constants
    |     LA = 1;
    |     LB = 1;
    |     L1 = LA/2;
    |     L2 = LB/2;
    |     % Damping Coefficents
    |     c1 = 2;
    |     c2 = 2;
    |     % Bar Mass Inertias
    |     I1 = 0.4167;
    |     I2 = 0.4167;
    |     % Gravity
    |     g = 10;
    | 
    |     yf = LA*cos(sp(1,1)) + LB*cos(sp(1,1)+sp(1,2));
    |     if((q(8)^2-2*g*(yf-q(4)))>=0)
    |         t = (q(8) + sqrt(q(8)^2-2*get*(yf-q(4))))/g;
    |     else
    |         t = 0.005;
    |     end
    | end

== matlab function PlanerizerTest03/Hip Position Function ==
  data: Pmux input; Pmux_out output
function Pmux_out  = Hip_Position(Pmux)
    % Pmux Planerizer encoder data
    %       [P(phi_1),P(phi_dot_1),P(phi_1),P(phi_dot_1)]

    ho = .4;
    lo = 1.85;
    
    phi   = Pmux(1);
    x     = lo*Pmux(1);
    y     = ho + lo*sin(Pmux(2));
    x_dot = lo*Pmux(3);
    y_dot = lo*Pmux(4)*cos(Pmux(2));

    Pmux_out = [phi x y x_dot y_dot];

== matlab function PlanerizerTest03/ID2 Write Knee Data/floats -> bytes ==
  data: position input; b output uint8 size=8; velocity input; K_p input; K_d input; T_ff input
function b = fcn(position, velocity, K_p, K_d, T_ff)

P_MIN  =-95.5;  % [rad]
P_MAX  = 95.5;  % [rad]
V_MIN  =-45;    % [rad/s] 30 to 45
V_MAX  = 45;    % [rad/s]
KP_MIN = 0;     % [Nm/rad]
KP_MAX = 500;   % [Nm/rad]
KD_MIN = 0;     % [Nm*s/rad
KD_MAX = 5;     % [Nm*s/rad
T_MIN  =-18;    % [Nm]
T_MAX  = 18;    % [Nm]

position = floor((max(min(position,P_MAX) ,P_MIN)  - P_MIN )*65535/(P_MAX  - P_MIN));
velocity = floor((max(min(velocity,V_MAX) ,V_MIN)  - V_MIN )*4095 /(V_MAX  - V_MIN));
K_p      = floor((max(min(K_p     ,KP_MAX),KP_MIN) - KP_MIN)*4095 /(KP_MAX - KP_MIN));
K_d      = floor((max(min(K_d     ,V_MAX) ,V_MIN)  - KD_MIN)*4095 /(KD_MAX - KD_MIN));
T_ff     = floor((max(min(T_ff    ,V_MAX) ,V_MIN)  - T_MIN )*4095 /(T_MAX  - T_MIN));

p  = dec2bin(position);
p  = [repmat('0', 1, 16-length(p)),p];
v  = dec2bin(velocity);
v  = [repmat('0', 1, 12-length(v)),v];
kp = dec2bin(K_p);
kp  = [repmat('0', 1, 12-length(kp)),kp];
kd = dec2bin(K_d);
kd  = [repmat('0', 1, 12-length(kd)),kd];
t  = dec2bin(T_ff);
t  = [repmat('0', 1, 12-length(t)),t];

B = repmat('0', 8, 8);

B(1,:) = p(1:8);
B(2,:) = p(9:16);
B(3,:) = v(1:8);
B(4,:) = [v(9:12),kp(1:4)];
B(5,:) = kp(5:12);
B(6,:) = kd(1:8);
B(7,:) = [kd(9:12),t(1:4)];
B(8,:) = t(5:12);

B  = bin2dec(B);

b = uint8(B);
